simulink model "gm_uz_ssi_interface_2025b"  (R2025b)
settings: Solver=FixedStepDiscrete  StartTime=0.0  StopTime=0.005  RelTol=1e-3
undefined symbols (not defined in the file or in its folder): binary_or_gray, bit_sum, delay_first_clk_on_off, f_ADC, f_clock, PLL, ssi_clk_divider, ssi_encoder_bit_width_multi_turn, ssi_encoder_bit_width_single_turn, ssi_encoder_number_of_status_bits, t_ADC, t_clock, XData
libraries: hdlmdlgenlib x104, hdlsllib x90, simulink x33, simulink_extras x7
(part 2 of 4)

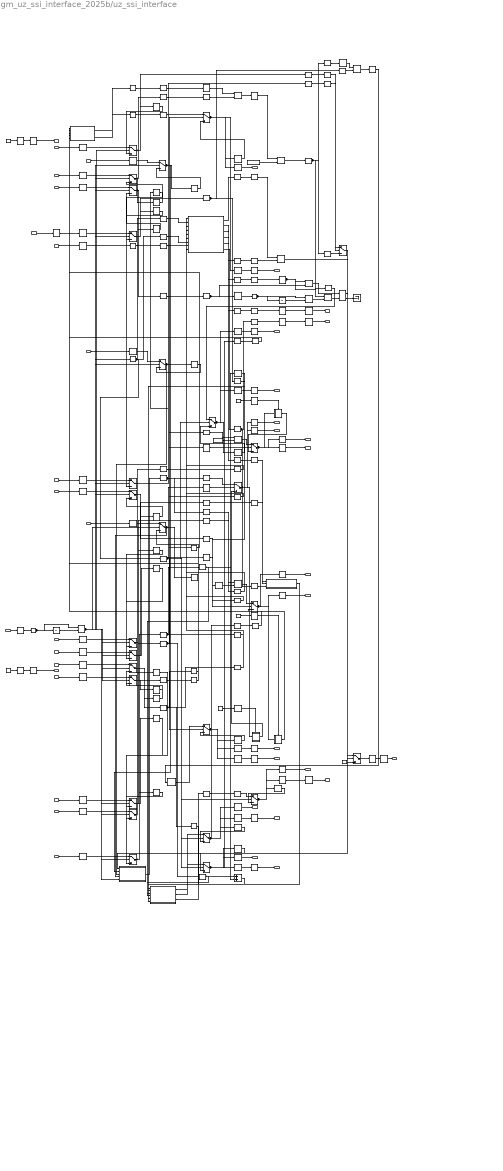
== system gm_uz_ssi_interface_2025b/uz_ssi_interface ==
  note: U(k)
  note: Edge
  note: U(k)
  note: Edge
  note: raw position with encoder offset and aligned wrap for ST and MT position
  note: Processing of raw position data
  note: mech speed SI to el speed SI
  note: decode position and slice data
  note: mech speed SI to el speed SI
  note: SI electrical position
  note: mech speed SI to mech speed RPM
  note: SI mech position to mech speed SI
  note: Acquisition of raw position data from the SSI absolute encoder
  note: ST mech position to SI mech position
  note: pull clk high when disabled
  note: enable logic for clock: turns on and off clk only between transmissions
  ssi_clk_divider_AXI : Inport  OutDataTypeStr=uint32  PortDimensions=1  SampleTime=1e-08
  ssi_encoder_bit_width_single_turn_AXI : Inport  Port=2  OutDataTypeStr=uint32  PortDimensions=1  SampleTime=1e-08
  ssi_encoder_bit_width_multi_turn_AXI : Inport  Port=3  OutDataTypeStr=uint32  PortDimensions=1  SampleTime=1e-08
  ssi_encoder_number_of_status_bits_AXI : Inport  Port=4  OutDataTypeStr=uint32  PortDimensions=1  SampleTime=1e-08
  delay_first_clk_on_off_AXI : Inport  Port=5  OutDataTypeStr=boolean  PortDimensions=1  SampleTime=1e-08
  pos_is_binary_or_gray_AXI : Inport  Port=6  OutDataTypeStr=boolean  PortDimensions=1  SampleTime=1e-08
  ssi_data_in : Inport  Port=7  OutDataTypeStr=boolean  PortDimensions=1  SampleTime=1e-08
  ssi_com_enable_AXI : Inport  Port=8  OutDataTypeStr=boolean  PortDimensions=1  SampleTime=1e-08
  trigger_ssi_read : Inport  Port=9  OutDataTypeStr=boolean  PortDimensions=1  SampleTime=1e-08
  reciprocal_bit_width_single_turn_AXI : Inport  Port=10  OutDataTypeStr=fixdt(0, 27, 27)  PortDimensions=1  SampleTime=1e-08
  t_sample_AXI : Inport  Port=11  OutDataTypeStr=fixdt(0, 18, 24)  PortDimensions=1  SampleTime=1e-08
  kp_pll_AXI : Inport  Port=12  OutDataTypeStr=fixdt(0, 18, 5)  PortDimensions=1  SampleTime=1e-08
  ki_pll_AXI : Inport  Port=13  OutDataTypeStr=fixdt(0, 18, 0)  PortDimensions=1  SampleTime=1e-08
  debug_off_on_AXI : Inport  Port=14  OutDataTypeStr=boolean  PortDimensions=1  SampleTime=1e-08
  position_mech_SI_debug_in_AXI : Inport  Port=15  OutDataTypeStr=fixdt(0, 27, 24)  PortDimensions=1  SampleTime=1e-08
  machine_polepairs_AXI : Inport  Port=16  OutDataTypeStr=uint32  PortDimensions=1  SampleTime=1e-08
  position_mech_offset_ticks_AXI : Inport  Port=17  OutDataTypeStr=int32  PortDimensions=1  SampleTime=1e-08
  sampling_delay_clk_ticks_AXI : Inport  Port=18  OutDataTypeStr=uint32  PortDimensions=1  SampleTime=1e-08
  AND : Logic  AllPortsSameDT=off  OutDataTypeStr=boolean  SampleTime=1e-08
  AND1 : Logic  AllPortsSameDT=off  OutDataTypeStr=boolean  SampleTime=1e-08
  Constant : Constant  Value=6.283172607421875  OutDataTypeStr=fixdt(0, 18, 15)  SampleTime=1e-08
  Constant1 : Constant  OutDataTypeStr=boolean  SampleTime=1e-08
  Constant3 : Constant  Value=0  OutDataTypeStr=boolean  SampleTime=1e-08
  Constant4 : Constant  Value=9.54931640625  OutDataTypeStr=fixdt(0, 18, 14)  SampleTime=1e-08
  Constant5 : Constant  OutDataTypeStr=boolean  SampleTime=1e-08
  Data Type Conversion : DataTypeConversion  OutDataTypeStr=uint8  SampleTime=1e-08  SaturateOnIntegerOverflow=off  RndMeth=Floor
  Data Type Conversion1 : DataTypeConversion  OutDataTypeStr=int32  SampleTime=1e-08  SaturateOnIntegerOverflow=off  RndMeth=Floor
  Delay{,4..5,7..8,10..11,13,15..20,22,24,26..27,29,33..34,37,39..43,46,48,50..52,54..58,62,127,129} (40 alike) : Delay  DelayLength=double(1)  InitialCondition=0  SampleTime=1e-08
  Delay Input1 : UnitDelay  SampleTime=1e-08
  Delay Input11 : UnitDelay  SampleTime=1e-08
  Delay1 : Delay  DelayLength=double(1)  InitialCondition=13  SampleTime=1e-08
  Delay{2..3,6,9,12,21,23,25,28,30,32,36,38,45,47,49,53,64} (18 alike) : Delay  DelayLength=double(2)  InitialCondition=0  SampleTime=1e-08
  Delay14 : Delay  DelayLength=double(1)  InitialCondition=1  SampleTime=1e-08
  Delay31 : Delay  DelayLength=double(1)  InitialCondition=25  SampleTime=1e-08
  Delay35 : Delay  DelayLength=double(1)  InitialCondition=1  SampleTime=1e-08
  Delay44 : Delay  DelayLength=double(1)  InitialCondition=12  SampleTime=1e-08
  Delay59_controlled : Subsystem
  Delay60_controlled : Subsystem
  Delay61_controlled : Subsystem
  FixPt Relational Operator : RelationalOperator  Operator=>  OutDataTypeStr=boolean  SampleTime=1e-08  InputSameDT=off
  FixPt Relational Operator1 : RelationalOperator  Operator=>  OutDataTypeStr=boolean  SampleTime=1e-08  InputSameDT=off
  From{,1..14,16..25,27..32,35..40,42..45} (41 alike) : hdlmdlgenlib/Buffer
  Goto{,1,3..12,14..29} (28 alike) : hdlmdlgenlib/Buffer
  Gray_code_to_binary : Subsystem
  NOT : Logic  Operator=NOT  Inputs=1  AllPortsSameDT=off  OutDataTypeStr=boolean  SampleTime=1e-08
  NOT1 : Logic  Operator=NOT  Inputs=1  AllPortsSameDT=off  OutDataTypeStr=boolean  SampleTime=1e-08
  OR : Logic  Operator=OR  AllPortsSameDT=off  OutDataTypeStr=boolean  SampleTime=1e-08
  Positive : simulink/Logic and Bit Operations/Compare To Constant  relop=>  const=double(0)  OutDataTypeStr=boolean
  Positive1 : simulink/Logic and Bit Operations/Compare To Constant  relop=>  const=double(0)  OutDataTypeStr=boolean
  Product : Product  Inputs=**  OutDataTypeStr=fixdt(0, 27, 24)  SampleTime=1e-08
  Product1 : Product  Inputs=**  OutDataTypeStr=fixdt(1, 27, 12)  SampleTime=1e-08
  Product2 : Product  Inputs=**  OutDataTypeStr=fixdt(1, 27, 12)  SampleTime=1e-08
  Product4 : Product  Inputs=**  OutDataTypeStr=fixdt(0, 27, 20)  SampleTime=1e-08
  Product7 : Product  Inputs=**  OutDataTypeStr=fixdt(0, 27, 24)  SampleTime=1e-08
  S-R Flip-Flop1 : simulink_extras/Flip Flops/S-R Flip-Flop  initial_condition=0
  S-R Flip-Flop1_inst_term1 : Terminator
  Sum2 : Sum  OutDataTypeStr=int32  AccumDataTypeStr=fixdt(0, 33, 0)  SampleTime=1e-08
  Switch{1,6,13,15..16,19..21,31} (9 alike) : Switch  Criteria=u2 > Threshold  Threshold="fi(0,0,1,0,\"hex\",\"0\")"  OutDataTypeStr=uint32  SampleTime=1e-08  SaturateOnIntegerOverflow=off  InputSameDT=off
  Switch{9..10,22,26} (4 alike) : Switch  Criteria=u2 > Threshold  Threshold="fi(0,0,1,0,\"hex\",\"0\")"  OutDataTypeStr=fixdt(0, 27, 24)  SampleTime=1e-08  SaturateOnIntegerOverflow=off  InputSameDT=off
  Switch11 : Switch  Criteria=u2 > Threshold  Threshold="fi(0,0,1,0,\"hex\",\"0\")"  OutDataTypeStr=uint8  SampleTime=1e-08  SaturateOnIntegerOverflow=off  InputSameDT=off
  Switch12 : Switch  Criteria=u2 > Threshold  Threshold="fi(0,0,1,0,\"hex\",\"0\")"  OutDataTypeStr=int32  SampleTime=1e-08  SaturateOnIntegerOverflow=off  InputSameDT=off
  Switch{5,8,14,17..18} (5 alike) : Switch  Criteria=u2 > Threshold  Threshold="fi(0,0,1,0,\"hex\",\"0\")"  OutDataTypeStr=boolean  SampleTime=1e-08  SaturateOnIntegerOverflow=off  InputSameDT=off
  Switch2 : Switch  Criteria=u2 > Threshold  Threshold="fi(0,0,1,0,\"hex\",\"0\")"  OutDataTypeStr=fixdt(0, 27, 27)  SampleTime=1e-08  SaturateOnIntegerOverflow=off  InputSameDT=off
  Switch23 : Switch  Criteria=u2 > Threshold  Threshold="fi(0,0,1,0,\"hex\",\"0\")"  OutDataTypeStr=fixdt(1, 27, 16)  SampleTime=1e-08  SaturateOnIntegerOverflow=off  InputSameDT=off
  Switch24 : Switch  Criteria=u2 > Threshold  Threshold="fi(0,0,1,0,\"hex\",\"0\")"  OutDataTypeStr=fixdt(1, 27, 12)  SampleTime=1e-08  SaturateOnIntegerOverflow=off  InputSameDT=off
  Switch25 : Switch  Criteria=u2 > Threshold  Threshold="fi(0,0,1,0,\"hex\",\"0\")"  OutDataTypeStr=fixdt(1, 27, 12)  SampleTime=1e-08  SaturateOnIntegerOverflow=off  InputSameDT=off
  Switch3 : Switch  Criteria=u2 > Threshold  Threshold="fi(0,0,1,0,\"hex\",\"0\")"  OutDataTypeStr=fixdt(0, 18, 24)  SampleTime=1e-08  SaturateOnIntegerOverflow=off  InputSameDT=off
  Switch4 : Switch  Criteria=u2 > Threshold  Threshold="fi(0,0,1,0,\"hex\",\"0\")"  OutDataTypeStr=fixdt(0, 18, 5)  SampleTime=1e-08  SaturateOnIntegerOverflow=off  InputSameDT=off
  Switch7 : Switch  Criteria=u2 > Threshold  Threshold="fi(0,0,1,0,\"hex\",\"0\")"  OutDataTypeStr=fixdt(0, 18, 0)  SampleTime=1e-08  SaturateOnIntegerOverflow=off  InputSameDT=off
  delayMatch{,1..23} (24 alike) : Delay  DelayLength=double(1)  InitialCondition=0  SampleTime=1e-08
  position_to_speed_pll : Subsystem
  set_offset_to_raw_position_and_wrap : Subsystem
  slice_position_and_status : Subsystem
  ssi_communication : Subsystem
  stateControl : Constant  OutDataTypeStr=boolean  SampleTime=1e-08
  stateControl1 : Constant  OutDataTypeStr=boolean  SampleTime=1e-08
  stateControl2 : Constant  OutDataTypeStr=boolean  SampleTime=1e-08
  wrap_2pi : Subsystem
  ssi_clk : Outport  SampleTime=1e-08
  RW_clk : Outport  Port=2  SampleTime=1e-08
  RW_data : Outport  Port=3  SampleTime=1e-08
  ssi_transaction_done : Outport  Port=4  OutDataTypeStr=boolean  SampleTime=1e-08  LockScale=on
  position_raw_single_turn : Outport  Port=5  OutDataTypeStr=uint32  SampleTime=1e-08  LockScale=on
  position_raw_single_turn_AXI : Outport  Port=6  OutDataTypeStr=uint32  SampleTime=1e-08  LockScale=on
  position_raw_multi_turn : Outport  Port=7  OutDataTypeStr=uint32  SampleTime=1e-08  LockScale=on
  position_raw_multi_turn_AXI : Outport  Port=8  OutDataTypeStr=uint32  SampleTime=1e-08  LockScale=on
  status_raw : Outport  Port=9  OutDataTypeStr=uint32  SampleTime=1e-08  LockScale=on
  status_raw_AXI : Outport  Port=10  OutDataTypeStr=uint32  SampleTime=1e-08  LockScale=on
  ssi_data_out_SH : Outport  Port=11  SampleTime=1e-08
  position_mech_SI_single_turn : Outport  Port=12  SampleTime=1e-08
  position_mech_SI_single_turn_AXI : Outport  Port=13  SampleTime=1e-08
  position_el_SI : Outport  Port=14  SampleTime=1e-08
  position_el_SI_AXI : Outport  Port=15  SampleTime=1e-08
  position_multi_turn : Outport  Port=16  OutDataTypeStr=uint32  SampleTime=1e-08  LockScale=on
  position_multi_turn_AXI : Outport  Port=17  OutDataTypeStr=uint32  SampleTime=1e-08  LockScale=on
  speed_mech_SI : Outport  Port=18  SampleTime=1e-08
  speed_mech_SI_AXI : Outport  Port=19  SampleTime=1e-08
  speed_el_SI : Outport  Port=20  SampleTime=1e-08
  speed_el_SI_AXI : Outport  Port=21  SampleTime=1e-08
  speed_mech_rpm : Outport  Port=22  SampleTime=1e-08
  speed_mech_rpm_AXI : Outport  Port=23  SampleTime=1e-08
  wires:
  Goto24/1 -> From5/1
  Delay53/1 -> Switch18/1
  Switch31/1 -> Delay31/1, Goto7/1
  Delay38/1 -> Switch12/1
  Delay Input11/1 -> FixPt Relational Operator1/2
  Delay12/1 -> Switch20/1
  Delay13/1 -> Switch21/3
  delayMatch14/1 -> position_raw_multi_turn_AXI/1
  Switch21/1 -> delayMatch22/1, Delay13/1, Delay41/1
  Data Type Conversion/1 -> Switch11/1
  From13/1 -> Switch9/1
  delayMatch8/1 -> RW_clk/1
  Delay9/1 -> Switch2/1
  Delay14/1 -> Switch5/3
  Delay41/1 -> delayMatch23/1
  Delay42/1 -> delayMatch21/1
  Positive1/1 -> FixPt Relational Operator1/1, Delay Input11/1
  slice_position_and_status/2(pos_raw_mt) -> Switch16/1
  From19/1 -> Switch9/3
  Switch9/1 -> position_to_speed_pll/1(position_mech_SI)
  Delay30/1 -> Switch10/1
  Delay Input1/1 -> FixPt Relational Operator/2
  Switch26/1 -> Delay42/1, Delay40/1, Delay62/1
  delayMatch1/1 -> Switch23/2
  Goto4/1 -> From42/1
  Delay47/1 -> Switch14/1
  Delay46/1 -> Switch14/3
  Delay49/1 -> Switch15/1
  Positive/1 -> FixPt Relational Operator/1, Delay Input1/1
  Delay22/1 -> Switch4/3
  Switch4/1 -> Delay22/1, position_to_speed_pll/3(kp_pll)
  Product2/1 -> Switch24/1
  Product1/1 -> Switch25/1
  Goto8/1 -> From11/1
  Delay28/1 -> Switch8/1
  From24/1 -> ssi_communication/4(In4)
  delayMatch/1 -> Delay59_controlled/Enable
  OR/1 -> Switch17/1
  ki_pll_AXI/1 -> Delay25/1
  Gray_code_to_binary/1(ssi_pos_binary) -> slice_position_and_status/1(data)
  Delay23/1 -> Switch4/1
  ssi_communication/5(ssi_data_out) -> Goto19/1
  Switch24/1 -> Delay60_controlled/1(in0), Delay56/1, Delay57/1
  Delay59_controlled/1(out0) -> Switch23/3
  FixPt Relational Operator1/1 -> Switch7/2, Switch4/2, Goto22/1, Switch13/2, Switch5/2, Switch20/2, Switch14/2, Switch11/2, Switch2/2, Switch10/2, Switch8/2, Switch1/2, Switch3/2, Switch15/2, position_to_speed_pll/5(Trigger), Switch12/2, Switch31/2, Switch18/2
  Delay24/1 -> Switch7/3
  From30/1 -> Switch19/1
  debug_off_on_AXI/1 -> Delay28/1
  Delay44/1 -> Switch13/3
  Delay25/1 -> Switch7/1
  Goto21/1 -> From18/1
  Delay40/1 -> delayMatch20/1
  From10/1 -> delayMatch1/1, Switch6/2, Switch22/2, Switch26/2, delayMatch6/1, Switch21/2, Switch19/2, delayMatch4/1, Switch16/2
  From28/1 -> NOT/1
  Delay11/1 -> delayMatch19/1
  Delay33/1 -> speed_mech_rpm/1
  Goto15/1 -> From43/1, From35/1, From24/1
  FixPt Relational Operator/1 -> AND1/2
  Delay21/1 -> Switch3/1
  Delay10/1 -> delayMatch18/1
  delayMatch11/1 -> position_raw_single_turn/1
  Delay20/1 -> Switch3/3
  Delay29/1 -> Switch10/3
  Goto22/1 -> From38/1, From39/1, From10/1
  Goto3/1 -> From7/1
  Delay4/1 -> delayMatch8/1
  delayMatch20/1 -> position_el_SI/1
  wrap_2pi/1(output) -> Switch26/1
  Delay55/1 -> delayMatch16/1
  Delay51/1 -> delayMatch14/1
  Delay15/1 -> Switch6/3
  Switch13/1 -> Goto15/1, Delay44/1
  stateControl1/1 -> delayMatch3/1
  Switch19/1 -> delayMatch15/1, Delay54/1, Delay55/1
  delayMatch13/1 -> position_raw_multi_turn/1
  Goto9/1 -> From25/1, From37/1
  Delay5/1 -> Switch20/3
  Delay6/1 -> Switch5/1
  From37/1 -> slice_position_and_status/4(bit_width_status), Sum2/2, Data Type Conversion1/1
  Switch8/1 -> Goto8/1, Delay27/1
  Goto/1 -> From23/1, From44/1, From36/1
  Delay31/1 -> Switch31/3
  Delay45/1 -> Switch13/1
  Delay2/1 -> Switch1/1
  slice_position_and_status/3(raw_status) -> Goto20/1
  Delay64/1 -> Switch31/1
  Delay17/1 -> delayMatch17/1
  Delay16/1 -> delayMatch12/1
  Product4/1 -> Delay43/1
  position_mech_offset_ticks_AXI/1 -> Delay38/1
  Delay129/1 -> delayMatch10/1
  Delay7/1 -> delayMatch9/1
  Goto28/1 -> From12/1
  stateControl/1 -> delayMatch/1
  Delay127/1 -> delayMatch7/1
  stateControl2/1 -> delayMatch5/1
  Delay34/1 -> speed_mech_rpm_AXI/1
  delay_first_clk_on_off_AXI/1 -> Delay6/1
  Delay57/1 -> speed_el_SI_AXI/1
  Delay56/1 -> speed_el_SI/1
  Switch14/1 -> Delay46/1, Goto16/1
  Delay18/1 -> speed_mech_SI_AXI/1
  Delay19/1 -> speed_mech_SI/1
  delayMatch10/1 -> ssi_transaction_done/1
  delayMatch23/1 -> position_multi_turn_AXI/1
  delayMatch21/1 -> position_el_SI_AXI/1
  Switch22/1 -> Delay10/1, Delay58/1, Delay11/1
  delayMatch19/1 -> position_mech_SI_single_turn_AXI/1
  delayMatch18/1 -> position_mech_SI_single_turn/1
  delayMatch17/1 -> ssi_data_out_SH/1
  From12/1 -> Switch21/1
  delayMatch16/1 -> status_raw_AXI/1
  delayMatch12/1 -> position_raw_single_turn_AXI/1
  delayMatch9/1 -> RW_data/1
  delayMatch7/1 -> ssi_clk/1
  set_offset_to_raw_position_and_wrap/1(st_raw_with_offset_and_wrapped) -> Goto29/1
  Goto5/1 -> From6/1
  Delay43/1 -> wrap_2pi/1(input)
  machine_polepairs_AXI/1 -> Delay36/1
  Goto27/1 -> From45/1
  Goto23/1 -> From40/1
  Goto7/1 -> From4/1
  Goto20/1 -> From30/1
  ssi_communication/1(ssi_clk) -> Goto24/1
  Goto19/1 -> From29/1
  Switch5/1 -> Delay14/1, Goto1/1
  Delay39/1 -> Product4/1
  delayMatch2/1 -> Product2/2
  Goto6/1 -> From28/1
  Goto18/1 -> From27/1
  Goto26/1 -> From20/1
  Goto29/1 -> From2/1
  Goto10/1 -> From13/1
  Goto1/1 -> From1/1
  ssi_communication/6(ssi_transaction_done) -> Goto17/1
  Constant/1 -> Product7/2
  ssi_communication/4(ssi_data_raw) -> Goto21/1
  S-R Flip-Flop1/1 -> Switch17/2
  ssi_communication/3(ssi_clk_idle_levels) -> Goto23/1
  ssi_communication/2(ssi_clk_enb_out) -> Goto6/1
  Goto14/1 -> From21/1, From19/1, From22/1
  slice_position_and_status/1(pos_raw_st) -> Switch6/1
  set_offset_to_raw_position_and_wrap/2(mt_raw_with_offset_and_wrapped) -> Goto28/1
  From7/1 -> ssi_communication/8(ssi_data_in)
  Constant1/1 -> Delay4/1
  position_to_speed_pll/1(speed_mech_SI) -> Goto12/1
  ssi_com_enable_AXI/1 -> Delay53/1
  From36/1 -> slice_position_and_status/3(bit_width_st), Sum2/1
  delayMatch22/1 -> position_multi_turn/1
  Switch15/1 -> Delay48/1, Goto9/1
  delayMatch15/1 -> status_raw/1
  ssi_data_in/1 -> Delay3/1
  Constant3/1 -> Delay7/1
  Switch17/1 -> Delay127/1
  From27/1 -> AND/2, NOT1/1
  S-R Flip-Flop1/2 -> S-R Flip-Flop1_inst_term1/1
  Product7/1 -> Goto14/1
  From9/1 -> ssi_communication/9(sampling_delay_clk_ticks)
  Product/1 -> Delay26/1
  Switch16/1 -> delayMatch13/1, Goto26/1, Delay50/1, Delay51/1
  NOT1/1 -> Positive/1
  From8/1 -> Gray_code_to_binary/3(trigger)
  From6/1 -> Product/2
  AND/1 -> S-R Flip-Flop1/1
  From5/1 -> OR/1
  From40/1 -> OR/2
  ssi_clk_divider_AXI/1 -> Delay64/1
  From39/1 -> ssi_communication/7(trigger_ssi)
  From38/1 -> ssi_communication/2(ssi_clk_reset)
  From31/1 -> Product2/1
  From3/1 -> Switch23/1
  t_sample_AXI/1 -> Delay21/1
  Delay/1 -> Product/1
  From29/1 -> Delay17/1
  Switch25/1 -> Delay61_controlled/1(in0), Delay34/1, Delay33/1
  From22/1 -> Delay39/1
  From2/1 -> Delay/1
  From18/1 -> Gray_code_to_binary/1(ssi_data_raw)
  From17/1 -> Gray_code_to_binary/2(pos_is_binary_or_gray)
  From16/1 -> Product4/2
  From14/1 -> Product1/1
  From11/1 -> Switch9/2
  From1/1 -> ssi_communication/6(delay_first_clk_on_off)
  ssi_encoder_number_of_status_bits_AXI/1 -> Delay49/1
  From/1 -> Delay129/1
  Constant4/1 -> Product1/2
  Delay36/1 -> Data Type Conversion/1
  Delay32/1 -> Positive1/1
  Delay3/1 -> Goto3/1
  sampling_delay_clk_ticks_AXI/1 -> Delay12/1
  Delay26/1 -> Product7/1
  Constant5/1 -> Switch17/3
  Switch6/1 -> Goto4/1, Delay16/1, Delay15/1, delayMatch11/1
  AND1/1 -> S-R Flip-Flop1/2
  position_mech_SI_debug_in_AXI/1 -> Delay30/1
  kp_pll_AXI/1 -> Delay23/1
  reciprocal_bit_width_single_turn_AXI/1 -> Delay9/1
  trigger_ssi_read/1 -> Delay32/1
  pos_is_binary_or_gray_AXI/1 -> Delay47/1
  ssi_encoder_bit_width_multi_turn_AXI/1 -> Delay45/1
  ssi_encoder_bit_width_single_turn_AXI/1 -> Delay2/1
  Switch23/1 -> Delay59_controlled/1(in0), Delay19/1, Delay18/1
  Goto12/1 -> From31/1, From14/1, From3/1
  Sum2/1 -> slice_position_and_status/5(shift_val_mt)
  Goto11/1 -> From16/1, From32/1
  Goto17/1 -> From8/1, From/1
  Switch7/1 -> position_to_speed_pll/4(ki_pll), Delay24/1
  Switch3/1 -> position_to_speed_pll/2(t_sample), Delay20/1
  Switch20/1 -> Goto25/1, Delay5/1
  Switch2/1 -> Goto5/1, Delay8/1
  Switch18/1 -> Goto18/1, Delay52/1
  Switch1/1 -> Goto/1, Delay1/1
  Switch12/1 -> Goto27/1, Delay37/1
  NOT/1 -> AND1/1, AND/1
  Switch11/1 -> Goto11/1, Delay35/1
  Switch10/1 -> Goto10/1, Delay29/1
  Delay52/1 -> Switch18/3
  delayMatch6/1 -> Switch25/2
  Goto25/1 -> From9/1
  Goto16/1 -> From17/1
  delayMatch4/1 -> Switch24/2
  Delay8/1 -> Switch2/3
  delayMatch3/1 -> Delay60_controlled/Enable
  delayMatch5/1 -> Delay61_controlled/Enable
  Delay27/1 -> Switch8/3
  Data Type Conversion1/1 -> slice_position_and_status/6(shift_val_st)
  Delay1/1 -> Switch1/3
  Delay37/1 -> Switch12/3
  Delay60_controlled/1(out0) -> Switch24/3
  Delay50/1 -> Switch16/3
  From43/1 -> set_offset_to_raw_position_and_wrap/5(n1)
  Delay61_controlled/1(out0) -> Switch25/3
  Delay35/1 -> Switch11/3
  Delay48/1 -> Switch15/3
  Delay54/1 -> Switch19/3
  Delay58/1 -> Switch22/3
  Delay62/1 -> Switch26/3
  From4/1 -> ssi_communication/1(ssi_clk_divider)
  From20/1 -> set_offset_to_raw_position_and_wrap/1(mt_raw)
  From21/1 -> Switch22/1
  From25/1 -> ssi_communication/5(In5)
  From23/1 -> ssi_communication/3(In3)
  From44/1 -> set_offset_to_raw_position_and_wrap/2(n)
  From32/1 -> delayMatch2/1
  From35/1 -> slice_position_and_status/2(bit_width_mt)
  From42/1 -> set_offset_to_raw_position_and_wrap/3(st_raw)
  From45/1 -> set_offset_to_raw_position_and_wrap/4(In4)

== system gm_uz_ssi_interface_2025b/uz_ssi_interface/Delay59_controlled ==
  in0 : Inport  OutDataTypeStr=fixdt(1, 27, 16)  SampleTime=1e-08
  stateControl : EnablePort  OutDataTypeStr=boolean
  Delay59 : Delay  DelayLength=double(1)  InitialCondition=0  SampleTime=1e-08
  out0 : Outport  OutDataTypeStr=fixdt(1, 27, 16)  SampleTime=1e-08
  wires:
  in0/1 -> Delay59/1
  Delay59/1 -> out0/1

== system gm_uz_ssi_interface_2025b/uz_ssi_interface/Delay60_controlled ==
  in0 : Inport  OutDataTypeStr=fixdt(1, 27, 12)  SampleTime=1e-08
  stateControl : EnablePort  OutDataTypeStr=boolean
  Delay60 : Delay  DelayLength=double(1)  InitialCondition=0  SampleTime=1e-08
  out0 : Outport  OutDataTypeStr=fixdt(1, 27, 12)  SampleTime=1e-08
  wires:
  in0/1 -> Delay60/1
  Delay60/1 -> out0/1

== system gm_uz_ssi_interface_2025b/uz_ssi_interface/Delay61_controlled ==
  in0 : Inport  OutDataTypeStr=fixdt(1, 27, 12)  SampleTime=1e-08
  stateControl : EnablePort  OutDataTypeStr=boolean
  Delay61 : Delay  DelayLength=double(1)  InitialCondition=0  SampleTime=1e-08
  out0 : Outport  OutDataTypeStr=fixdt(1, 27, 12)  SampleTime=1e-08
  wires:
  in0/1 -> Delay61/1
  Delay61/1 -> out0/1

== system gm_uz_ssi_interface_2025b/uz_ssi_interface/Gray_code_to_binary ==
  ssi_data_raw : Inport  OutDataTypeStr=fixdt(0, 64, 0)  PortDimensions=1  SampleTime=1e-08
  pos_is_binary_or_gray : Inport  Port=2  OutDataTypeStr=boolean  PortDimensions=1  SampleTime=1e-08
  trigger : Inport  Port=3  OutDataTypeStr=boolean  PortDimensions=1  SampleTime=1e-08
  Delay : Delay  DelayLength=double(1)  InitialCondition=0  SampleTime=1e-08
  Delay2 : Delay  DelayLength=double(101)  InitialCondition=0  SampleTime=1e-08
  Delay6 : Delay  DelayLength=double(1)  InitialCondition=0  SampleTime=1e-08
  Switch : Switch  Criteria=u2 > Threshold  Threshold="fi(0,0,1,0,\"hex\",\"0\")"  OutDataTypeStr=fixdt(0, 64, 0)  SampleTime=1e-08  SaturateOnIntegerOverflow=off  InputSameDT=off
  gray_to_bin : Subsystem
  ssi_pos_binary : Outport  SampleTime=1e-08
  wires:
  ssi_data_raw/1 -> Delay/1, Delay2/1
  trigger/1 -> gray_to_bin/2(enb)
  Delay/1 -> gray_to_bin/1(gray)
  gray_to_bin/1(binary_out) -> Delay6/1
  pos_is_binary_or_gray/1 -> Switch/2
  Delay2/1 -> Switch/3
  Delay6/1 -> Switch/1
  Switch/1 -> ssi_pos_binary/1

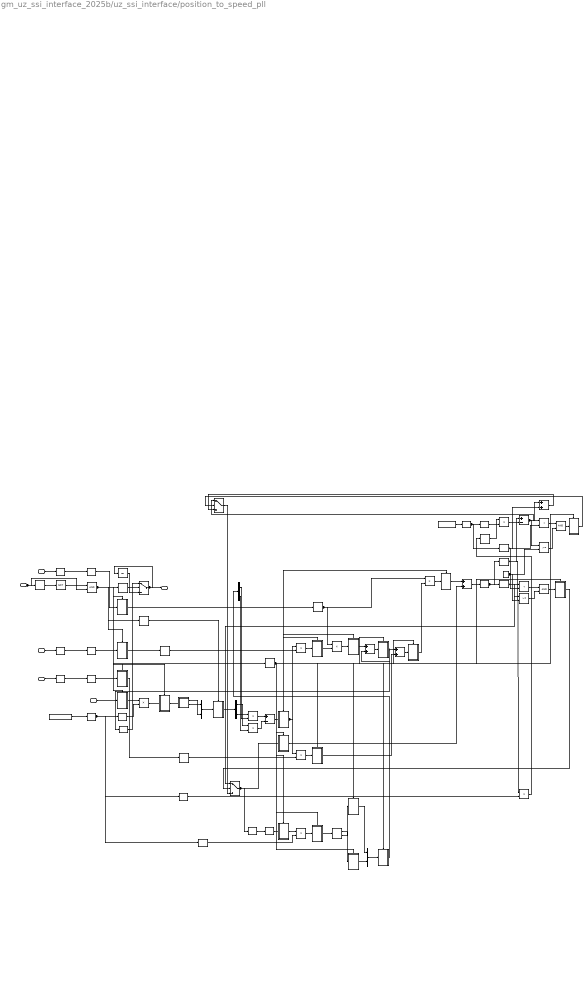
== system gm_uz_ssi_interface_2025b/uz_ssi_interface/position_to_speed_pll ==
  note: pi_controller
  note: +/- 198000
  note: -2 ... 2
  note: wrap 2pi
  note: <<1
  note: phase discriminator
  note: -1 ... 1
  note: pll
  note: -1 ... 1
  note: integrator
  note: 20
  note: +/- 1300
  note: remainder
  position_mech_SI : Inport  OutDataTypeStr=fixdt(0, 27, 24)  PortDimensions=1  SampleTime=1e-08
  t_sample : Inport  Port=2  OutDataTypeStr=fixdt(0, 18, 24)  PortDimensions=1  SampleTime=1e-08
  kp_pll : Inport  Port=3  OutDataTypeStr=fixdt(0, 18, 5)  PortDimensions=1  SampleTime=1e-08
  ki_pll : Inport  Port=4  OutDataTypeStr=fixdt(0, 18, 0)  PortDimensions=1  SampleTime=1e-08
  Trigger : Inport  Port=5  OutDataTypeStr=boolean  SampleTime=1e-08
  AND : Logic  AllPortsSameDT=off  OutDataTypeStr=boolean  SampleTime=1e-08
  AND1 : Logic  AllPortsSameDT=off  OutDataTypeStr=boolean  SampleTime=1e-08
  Constant1 : Constant  Value=0.1591548919677734375  OutDataTypeStr=fixdt(0, 18, 20)  SampleTime=1e-08
  Constant7 : Constant  Value=0  OutDataTypeStr=fixdt(0, 27, 24)  SampleTime=1e-08
  Constant8 : Constant  Value=6.283172607421875  OutDataTypeStr=fixdt(0, 18, 15)  SampleTime=1e-08
  Delay : Subsystem
      settings: MinAlgLoopOccurrences=on
  Delay1 : Subsystem
      settings: MinAlgLoopOccurrences=on
  Delay10 : Subsystem
      settings: MinAlgLoopOccurrences=on
  Delay11 : Subsystem
      settings: MinAlgLoopOccurrences=on
  Delay12 : Subsystem
      settings: MinAlgLoopOccurrences=on
  Delay13 : Subsystem
      settings: MinAlgLoopOccurrences=on
  Delay14 : Subsystem
      settings: MinAlgLoopOccurrences=on
  Delay18 : Subsystem
      settings: MinAlgLoopOccurrences=on
  Delay19 : Subsystem
      settings: MinAlgLoopOccurrences=on
  Delay2 : Subsystem
      settings: MinAlgLoopOccurrences=on
  Delay20 : Subsystem
      settings: MinAlgLoopOccurrences=on
  Delay21 : Subsystem
      settings: MinAlgLoopOccurrences=on
  Delay22 : Subsystem
      settings: MinAlgLoopOccurrences=on
  Delay23 : Subsystem
      settings: MinAlgLoopOccurrences=on
  Delay3 : Subsystem
      settings: MinAlgLoopOccurrences=on
  Delay4 : Subsystem
      settings: MinAlgLoopOccurrences=on
  Delay5 : Subsystem
      settings: MinAlgLoopOccurrences=on
  Delay6 : Subsystem
      settings: MinAlgLoopOccurrences=on
  Delay7 : Subsystem
      settings: MinAlgLoopOccurrences=on
  Delay8 : Subsystem
      settings: MinAlgLoopOccurrences=on
  Delay9 : Subsystem
      settings: MinAlgLoopOccurrences=on
  From{,1..6,11,13..15} (11 alike) : hdlmdlgenlib/Buffer
  Goto{,1..3,8,10..11} (7 alike) : hdlmdlgenlib/Buffer
  Product1 : Product  Inputs=**  OutDataTypeStr=fixdt(1, 27, 23)  SampleTime=1e-08
  Product10 : Product  Inputs=**  OutDataTypeStr=fixdt(1, 27, 20)  SampleTime=1e-08
  Product2 : Product  Inputs=**  OutDataTypeStr=fixdt(1, 27, 25)  SampleTime=1e-08
  Product3 : Product  Inputs=**  OutDataTypeStr=fixdt(1, 27, 25)  SampleTime=1e-08
  Product4 : Product  Inputs=**  OutDataTypeStr=fixdt(1, 27, 20)  SampleTime=1e-08
  Product5 : Product  Inputs=**  OutDataTypeStr=fixdt(1, 27, 8)  SampleTime=1e-08
  Product6 : Product  Inputs=**  OutDataTypeStr=fixdt(1, 27, 14)  SampleTime=1e-08
  Product7 : Product  Inputs=**  OutDataTypeStr=fixdt(1, 27, 23)  SampleTime=1e-08
  Product8 : Product  Inputs=**  OutDataTypeStr=fixdt(1, 27, 26)  SampleTime=1e-08
  Product9 : Product  Inputs=**  OutDataTypeStr=fixdt(1, 27, 20)  SampleTime=1e-08
  Relational Operator1 : RelationalOperator  Operator=<  OutDataTypeStr=boolean  SampleTime=1e-08  InputSameDT=off
  Relational Operator2 : RelationalOperator  OutDataTypeStr=boolean  SampleTime=1e-08  InputSameDT=off
  Relational Operator3 : RelationalOperator  Operator=<  OutDataTypeStr=boolean  SampleTime=1e-08  InputSameDT=off
  Relational Operator4 : RelationalOperator  OutDataTypeStr=boolean  SampleTime=1e-08  InputSameDT=off
  Sine HDL Optimized : Subsystem  mask(Sine and Cosine HDL optimized block){OutputFormula=sin(2*pi*u) and cos(2*pi*u), NumDataPoints=double(256), TableDataTypeStr=fixdt(0,26,20), SimulateLUTROMDelay=off}
      mask prompts: OutputFormula "Simulink:masks:OutputFormula_MP"; NumDataPoints "HDLShared:hdlshared:CosineHDL_Npts"; TableDataTypeStr "Simulink:blkprm_prompts:TABLE_UNIFIEDDATATYPE"; SimulateLUTROMDelay "HDLShared:hdlshared:CosineHDL_SimulateLUTDelay"
      mask help: Sine and Cosine HDL optimized block using quarter wave symmetry, and HDL friendly settings.
      mask init:
      | NumDataPoints = double(256);
      | OutputFormula = double(4);
      | SampleTime = double(-1);
      | SimulateLUTROMDelay = double(0);
      | TableDataTypeStr = fixdt(0,26,20);
      | curr_blk_name = 'uz_ssi_interface_2025b/uz_ssi_interface/position_to_speed_pll/Sine\nHDL Optimized';
      | sys_name = 'uz_ssi_interface_2025b/uz_ssi_interface/position_to_speed_pll';
      mask Help: helpview([docroot '/hdlcoder/helptargets.map'],'SineAndCosineHDL_Optimized');
      mask TypeOptions OutputFormula: sin(2*pi*u) | cos(2*pi*u) | exp(j*2*pi*u) | sin(2*pi*u) and cos(2*pi*u)
      mask Display:
      | port_label('input',1,'u')
      | port_label('output',1,'sin(2*pi*u)')
      | port_label('output',2,'cos(2*pi*u)')
      | xpos = 0.35;
      | yoffset = 0.5;
      | if ( SimulateLUTROMDelay )
      |   text(xpos,yoffset,'HDL (Z^{-1})','texmode','on')
      | else
      |    text(xpos,yoffset,'HDL')
      | end
  Sine HDL Optimized1 : Subsystem  mask(Sine and Cosine HDL optimized block){OutputFormula=sin(2*pi*u) and cos(2*pi*u), NumDataPoints=double(256), TableDataTypeStr=fixdt(0,26,20), SimulateLUTROMDelay=off}
      mask prompts: OutputFormula "Simulink:masks:OutputFormula_MP"; NumDataPoints "HDLShared:hdlshared:CosineHDL_Npts"; TableDataTypeStr "Simulink:blkprm_prompts:TABLE_UNIFIEDDATATYPE"; SimulateLUTROMDelay "HDLShared:hdlshared:CosineHDL_SimulateLUTDelay"
      mask help: Sine and Cosine HDL optimized block using quarter wave symmetry, and HDL friendly settings.
      mask init:
      | NumDataPoints = double(256);
      | OutputFormula = double(4);
      | SampleTime = double(-1);
      | SimulateLUTROMDelay = double(0);
      | TableDataTypeStr = fixdt(0,26,20);
      | curr_blk_name = 'uz_ssi_interface_2025b/uz_ssi_interface/position_to_speed_pll/Sine\nHDL Optimized1';
      | sys_name = 'uz_ssi_interface_2025b/uz_ssi_interface/position_to_speed_pll';
      mask Help: helpview([docroot '/hdlcoder/helptargets.map'],'SineAndCosineHDL_Optimized');
      mask TypeOptions OutputFormula: sin(2*pi*u) | cos(2*pi*u) | exp(j*2*pi*u) | sin(2*pi*u) and cos(2*pi*u)
      mask Display:
      | port_label('input',1,'u')
      | port_label('output',1,'sin(2*pi*u)')
      | port_label('output',2,'cos(2*pi*u)')
      | xpos = 0.35;
      | yoffset = 0.5;
      | if ( SimulateLUTROMDelay )
      |   text(xpos,yoffset,'HDL (Z^{-1})','texmode','on')
      | else
      |    text(xpos,yoffset,'HDL')
      | end
  Sum1 : Sum  Inputs=+-  OutDataTypeStr=fixdt(1, 27, 24)  AccumDataTypeStr=fixdt(1, 27, 24)  SampleTime=1e-08
  Sum2 : Sum  OutDataTypeStr=fixdt(1, 27, 16)  AccumDataTypeStr=fixdt(1, 32, 20)  SampleTime=1e-08
  Sum3 : Sum  OutDataTypeStr=fixdt(1, 27, 14)  AccumDataTypeStr=fixdt(1, 30, 16)  SampleTime=1e-08
  Sum4 : Sum  OutDataTypeStr=fixdt(1, 27, 23)  AccumDataTypeStr=fixdt(1, 31, 26)  SampleTime=1e-08
  Sum5 : Sum  Inputs=+-  OutDataTypeStr=fixdt(1, 27, 23)  AccumDataTypeStr=fixdt(1, 28, 23)  SampleTime=1e-08
  Sum6 : Sum  OutDataTypeStr=fixdt(1, 27, 23)  AccumDataTypeStr=fixdt(1, 28, 23)  SampleTime=1e-08
  Switch3 : Switch  Criteria=u2 > Threshold  Threshold="fi(0,0,1,0,\"hex\",\"0\")"  OutDataTypeStr=fixdt(1, 27, 23)  SampleTime=1e-08  SaturateOnIntegerOverflow=off  InputSameDT=off
  Switch4 : Switch  Criteria=u2 > Threshold  Threshold="fi(0,0,1,0,\"hex\",\"0\")"  OutDataTypeStr=fixdt(1, 27, 23)  SampleTime=1e-08  SaturateOnIntegerOverflow=off  InputSameDT=off
  Trigger_delay : Delay  DelayLength=double(1)  InitialCondition=0
  Trigger_delayed_inverted_and_Trigger : Logic  AllPortsSameDT=off  OutDataTypeStr=boolean  SampleTime=1e-08
  delayMatch{,1..5} (6 alike) : Delay  DelayLength=double(1)  InitialCondition=0
  fixed_point_floor : Subsystem
  mux : Mux  Inputs=2
  mux1 : Mux  Inputs=2
  not_Trigger_delayed : Logic  Operator=NOT  Inputs=1  AllPortsSameDT=off  OutDataTypeStr=boolean  SampleTime=1e-08
  omega_mechbypassMux : Switch  Criteria=u2 ~= 0  Threshold=double(0)  OutDataTypeStr=fixdt(1, 27, 16)  SampleTime=1e-08  SaturateOnIntegerOverflow=off  InputSameDT=off
  out0_bypass : UnitDelay  InitialCondition="fi(0,1,27,16,\"hex\",\"0000000\")"  SampleTime=1e-08
  t : Demux  Outputs=2
  t1 : Demux  Outputs=2
  t2 : hdlmdlgenlib/Buffer
  speed_mech_SI : Outport  SampleTime=1e-08  InitialOutput=[0]
  wires:
  Goto2/1 -> From2/1
  Delay14/1(out0) -> Sine HDL Optimized1/1(u)
  ki_pll/1 -> Goto2/1
  delayMatch5/1 -> omega_mechbypassMux/2
  Trigger/1 -> Trigger_delayed_inverted_and_Trigger/2, Trigger_delay/1
  Delay3/1(out0) -> Sum3/2
  From4/1 -> Product7/2
  delayMatch/1 -> Delay1/Enable
  t_sample/1 -> Goto/1
  Delay4/1(out0) -> Sum2/1
  Trigger_delay/1 -> not_Trigger_delayed/1
  Trigger_delayed_inverted_and_Trigger/1 -> Delay13/Enable, delayMatch/1, Delay7/Enable, delayMatch1/1, Delay6/Enable, delayMatch5/1, Delay14/Enable, Delay8/Enable
  kp_pll/1 -> Goto1/1
  not_Trigger_delayed/1 -> Trigger_delayed_inverted_and_Trigger/1
  Goto/1 -> From/1
  From3/1 -> Delay11/1(in0)
  Goto1/1 -> From1/1
  Delay5/1(out0) -> Product4/2
  Constant1/1 -> Goto3/1
  omega_mechbypassMux/1 -> out0_bypass/1, speed_mech_SI/1
  out0_bypass/1 -> omega_mechbypassMux/3
  From/1 -> Delay6/1(in0)
  From2/1 -> Delay7/1(in0)
  From1/1 -> Delay8/1(in0)
  Delay1/1(out0) -> t/1
  Delay19/1(out0) -> Sum4/2
  position_mech_SI/1 -> Delay13/1(in0)
  From15/1 -> Sum5/1, Product7/1
  Goto3/1 -> From4/1, From6/1, From5/1
  Sine HDL Optimized1/1(x) -> mux/2
  Delay6/1(out0) -> delayMatch3/1
  Product5/1 -> Delay5/1(in0)
  Delay7/1(out0) -> delayMatch4/1
  Product3/1 -> Sum1/1
  Delay8/1(out0) -> delayMatch2/1
  From13/1 -> Relational Operator3/2, Sum6/2, Relational Operator1/2
  Delay11/1(out0) -> Product9/1
  Delay23/1(out0) -> mux1/1
  Delay13/1(out0) -> Product10/1
  Switch3/1 -> Delay19/1(in0), Goto8/1
  From6/1 -> Product10/2
  t2/1 -> omega_mechbypassMux/1
  Product10/1 -> Delay14/1(in0)
  delayMatch4/1 -> Product5/2
  Sine HDL Optimized1/2(y) -> mux/1
  delayMatch3/1 -> Product8/1, Product4/1
  delayMatch2/1 -> Product6/2
  Delay12/1(out0) -> Sine HDL Optimized/1(u)
  Product2/1 -> Sum1/2
  mux/1 -> Delay1/1(in0)
  From5/1 -> Product9/2
  Switch4/1 -> Switch3/3
  t1/2 -> Product2/2
  t1/1 -> Product3/2
  t/2 -> Product3/1
  t/1 -> Product2/1
  Goto8/1 -> From3/1
  delayMatch1/1 -> Delay2/Enable, Delay11/Enable, Delay9/Enable, Delay10/Enable, Delay18/Enable, Delay5/Enable, Delay4/Enable, Delay20/Enable, Delay21/Enable, Delay22/Enable, Delay23/Enable, Delay19/Enable, Delay3/Enable, Delay/Enable, Delay12/Enable
  Sum1/1 -> Delay2/1(in0)
  Delay2/1(out0) -> Product6/1, Product5/1
  Product6/1 -> Delay3/1(in0)
  Product9/1 -> Delay12/1(in0)
  Sine HDL Optimized/1(x) -> Delay22/1(in0)
  Product4/1 -> Delay4/1(in0)
  Sine HDL Optimized/2(y) -> Delay23/1(in0)
  Delay20/1(out0) -> Switch4/2
  Delay22/1(out0) -> mux1/2
  Sum2/1 -> Delay/1(in0)
  mux1/1 -> Delay18/1(in0)
  Delay/1(out0) -> Sum2/2, t2/1, Sum3/1
  Delay18/1(out0) -> t1/1
  Sum3/1 -> Delay9/1(in0)
  Delay9/1(out0) -> Product8/2
  Product8/1 -> Delay10/1(in0)
  Constant8/1 -> Goto11/1
  Delay10/1(out0) -> Sum4/1
  Goto11/1 -> From13/1, From14/1
  Sum4/1 -> Goto10/1
  From14/1 -> Product1/2
  fixed_point_floor/1(y) -> Product1/1
  Goto10/1 -> From15/1, From11/1
  Product1/1 -> Sum5/2
  Constant7/1 -> Relational Operator4/2, Relational Operator2/2
  From11/1 -> Switch3/1, Relational Operator2/1, Relational Operator1/1
  Sum5/1 -> Switch4/1, Sum6/1, Relational Operator4/1, Relational Operator3/1
  Relational Operator1/1 -> AND/1
  Relational Operator2/1 -> AND/2
  Product7/1 -> fixed_point_floor/1(x)
  Sum6/1 -> Switch4/3
  Relational Operator3/1 -> AND1/1
  Relational Operator4/1 -> AND1/2
  AND/1 -> Delay21/1(in0)
  AND1/1 -> Delay20/1(in0)
  Delay21/1(out0) -> Switch3/2

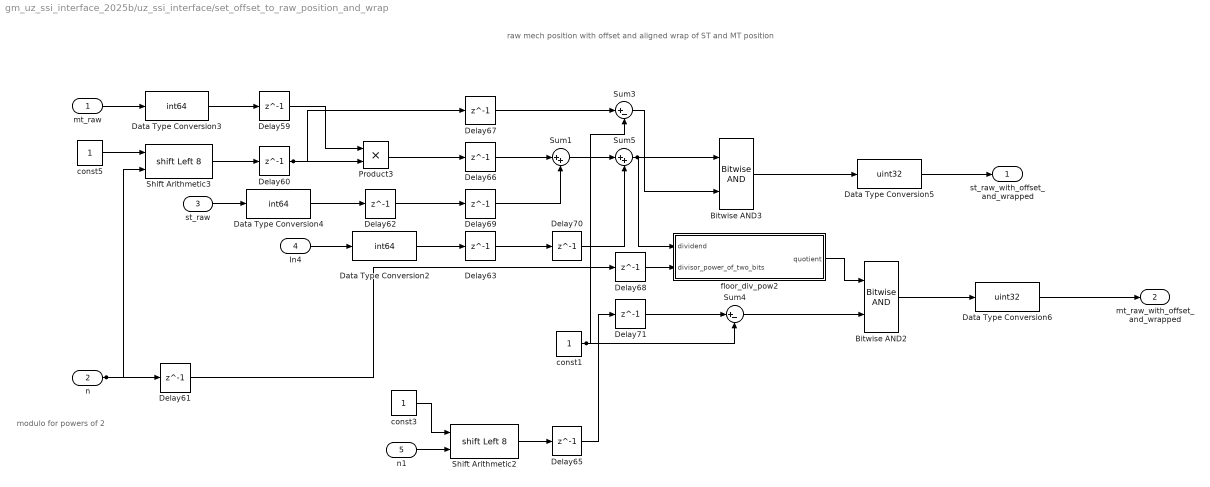
== system gm_uz_ssi_interface_2025b/uz_ssi_interface/set_offset_to_raw_position_and_wrap ==
  note: modulo for powers of 2
  note: raw mech position with offset and aligned wrap of ST and MT position
  mt_raw : Inport  OutDataTypeStr=uint32  PortDimensions=1  SampleTime=1e-08
  n : Inport  Port=2  OutDataTypeStr=uint32  PortDimensions=1  SampleTime=1e-08
  st_raw : Inport  Port=3  OutDataTypeStr=uint32  PortDimensions=1  SampleTime=1e-08
  In4 : Inport  Port=4  OutDataTypeStr=int32  PortDimensions=1  SampleTime=1e-08
  n1 : Inport  Port=5  OutDataTypeStr=uint32  PortDimensions=1  SampleTime=1e-08
  Bitwise AND2 : simulink/Logic and Bit Operations/Bitwise Operator  logicop=AND  UseBitMask=off  NumInputPorts=2  BitMask=bin2dec('11011001')  BitMaskRealWorld=Stored Integer
      settings: LibrarySourceBlock=|
      | simulink/Quick Insert/Logic and Bit
      | Operations/Bitwise AND
  Bitwise AND3 : simulink/Logic and Bit Operations/Bitwise Operator  logicop=AND  UseBitMask=off  NumInputPorts=2  BitMask=bin2dec('11011001')  BitMaskRealWorld=Stored Integer
      settings: LibrarySourceBlock=|
      | simulink/Quick Insert/Logic and Bit
      | Operations/Bitwise AND
  Data Type Conversion2 : DataTypeConversion  OutDataTypeStr=int64  SaturateOnIntegerOverflow=off  RndMeth=Floor
  Data Type Conversion3 : DataTypeConversion  OutDataTypeStr=int64  SaturateOnIntegerOverflow=off  RndMeth=Floor
  Data Type Conversion4 : DataTypeConversion  OutDataTypeStr=int64  SaturateOnIntegerOverflow=off  RndMeth=Floor
  Data Type Conversion5 : DataTypeConversion  OutDataTypeStr=uint32  SaturateOnIntegerOverflow=off  RndMeth=Floor
  Data Type Conversion6 : DataTypeConversion  OutDataTypeStr=uint32  SaturateOnIntegerOverflow=off  RndMeth=Floor
  Delay{59..63,65..71} (12 alike) : Delay  DelayLength=1  InitialCondition=0
  Product3 : Product  OutDataTypeStr=int64
  Shift Arithmetic2 : ArithShift  BitShiftNumberSource=Input port  BitShiftNumber=8  BitShiftDirection=Left
      settings: InputPortMap=u0,p1
  Shift Arithmetic3 : ArithShift  BitShiftNumberSource=Input port  BitShiftNumber=8  BitShiftDirection=Left
      settings: InputPortMap=u0,p1
  Sum1 : Sum  Inputs=|++  OutDataTypeStr=int64
  Sum3 : Sum  Inputs=|+-  OutDataTypeStr=int64
  Sum4 : Sum  Inputs=|+-  OutDataTypeStr=int64
  Sum5 : Sum  Inputs=|++  OutDataTypeStr=int64
  const1 : Constant  OutDataTypeStr=int64  SampleTime=t_clock
  const3 : Constant  OutDataTypeStr=int64  SampleTime=t_clock
  const5 : Constant  OutDataTypeStr=int64  SampleTime=t_clock
  floor_div_pow2 : Subsystem
  st_raw_with_offset_and_wrapped : Outport  SampleTime=1e-08
  mt_raw_with_offset_and_wrapped : Outport  Port=2  SampleTime=1e-08
  wires:
  Delay69/1 -> Sum1/2
  Delay60/1 -> Delay67/1, Product3/2
  Delay61/1 -> Delay68/1
  mt_raw/1 -> Data Type Conversion3/1
  Shift Arithmetic3/1 -> Delay60/1
  const5/1 -> Shift Arithmetic3/1
  Data Type Conversion6/1 -> mt_raw_with_offset_and_wrapped/1
  n/1 -> Delay61/1, Shift Arithmetic3/2
  Data Type Conversion4/1 -> Delay62/1
  Data Type Conversion3/1 -> Delay59/1
  st_raw/1 -> Data Type Conversion4/1
  Sum4/1 -> Bitwise AND2/2
  Delay59/1 -> Product3/1
  In4/1 -> Data Type Conversion2/1
  Product3/1 -> Delay66/1
  Sum1/1 -> Sum5/1
  Delay62/1 -> Delay69/1
  const3/1 -> Shift Arithmetic2/1
  Data Type Conversion2/1 -> Delay63/1
  n1/1 -> Shift Arithmetic2/2
  Delay67/1 -> Sum3/1
  Delay66/1 -> Sum1/1
  Sum3/1 -> Bitwise AND3/2
  Delay63/1 -> Delay70/1
  Shift Arithmetic2/1 -> Delay65/1
  Delay70/1 -> Sum5/2
  const1/1 -> Sum3/2, Sum4/2
  Delay65/1 -> Delay71/1
  Sum5/1 -> Bitwise AND3/1, floor_div_pow2/1(dividend)
  Delay68/1 -> floor_div_pow2/2(divisor_power_of_two_bits)
  Delay71/1 -> Sum4/1
  Bitwise AND3/1 -> Data Type Conversion5/1
  floor_div_pow2/1(quotient) -> Bitwise AND2/1
  Data Type Conversion5/1 -> st_raw_with_offset_and_wrapped/1
  Bitwise AND2/1 -> Data Type Conversion6/1

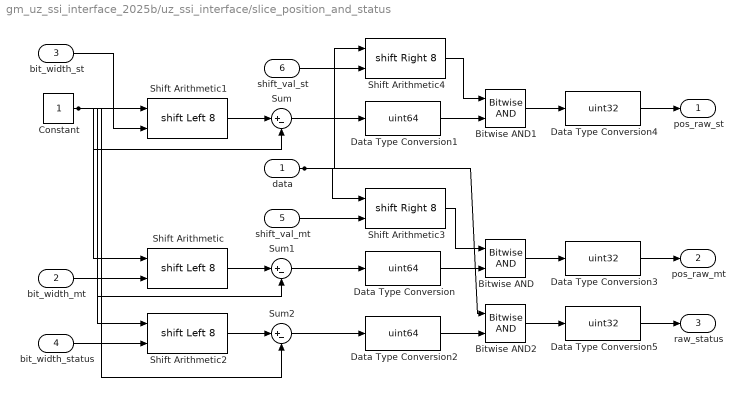
== system gm_uz_ssi_interface_2025b/uz_ssi_interface/slice_position_and_status ==
  data : Inport  OutDataTypeStr=fixdt(0, 64, 0)  PortDimensions=1  SampleTime=1e-08
  bit_width_mt : Inport  Port=2  OutDataTypeStr=uint32  PortDimensions=1  SampleTime=1e-08
  bit_width_st : Inport  Port=3  OutDataTypeStr=uint32  PortDimensions=1  SampleTime=1e-08
  bit_width_status : Inport  Port=4  OutDataTypeStr=uint32  PortDimensions=1  SampleTime=1e-08
  shift_val_mt : Inport  Port=5  OutDataTypeStr=int32  PortDimensions=1  SampleTime=1e-08
  shift_val_st : Inport  Port=6  OutDataTypeStr=int32  PortDimensions=1  SampleTime=1e-08
  Bitwise AND : simulink/Logic and Bit Operations/Bitwise Operator  logicop=AND  UseBitMask=off  NumInputPorts=2  BitMask=bin2dec('11011001')  BitMaskRealWorld=Stored Integer
      settings: LibrarySourceBlock=|
      | simulink/Quick Insert/Logic and Bit
      | Operations/Bitwise AND
  Bitwise AND1 : simulink/Logic and Bit Operations/Bitwise Operator  logicop=AND  UseBitMask=off  NumInputPorts=2  BitMask=bin2dec('11011001')  BitMaskRealWorld=Stored Integer
      settings: LibrarySourceBlock=|
      | simulink/Quick Insert/Logic and Bit
      | Operations/Bitwise AND
  Bitwise AND2 : simulink/Logic and Bit Operations/Bitwise Operator  logicop=AND  UseBitMask=off  NumInputPorts=2  BitMask=bin2dec('11011001')  BitMaskRealWorld=Stored Integer
      settings: LibrarySourceBlock=|
      | simulink/Quick Insert/Logic and Bit
      | Operations/Bitwise AND
  Constant : Constant  OutDataTypeStr=uint32  SampleTime=t_clock
  Data Type Conversion : DataTypeConversion  OutDataTypeStr=uint64  SaturateOnIntegerOverflow=off  RndMeth=Floor
  Data Type Conversion1 : DataTypeConversion  OutDataTypeStr=uint64  SaturateOnIntegerOverflow=off  RndMeth=Floor
  Data Type Conversion2 : DataTypeConversion  OutDataTypeStr=uint64  SaturateOnIntegerOverflow=off  RndMeth=Floor
  Data Type Conversion3 : DataTypeConversion  OutDataTypeStr=uint32  SaturateOnIntegerOverflow=off  RndMeth=Floor
  Data Type Conversion4 : DataTypeConversion  OutDataTypeStr=uint32  SaturateOnIntegerOverflow=off  RndMeth=Floor
  Data Type Conversion5 : DataTypeConversion  OutDataTypeStr=uint32  SaturateOnIntegerOverflow=off  RndMeth=Floor
  Shift Arithmetic : ArithShift  BitShiftNumberSource=Input port  BitShiftNumber=8  BitShiftDirection=Left
      settings: InputPortMap=u0,p1
  Shift Arithmetic1 : ArithShift  BitShiftNumberSource=Input port  BitShiftNumber=8  BitShiftDirection=Left
      settings: InputPortMap=u0,p1
  Shift Arithmetic2 : ArithShift  BitShiftNumberSource=Input port  BitShiftNumber=8  BitShiftDirection=Left
      settings: InputPortMap=u0,p1
  Shift Arithmetic3 : ArithShift  BitShiftNumberSource=Input port  BitShiftNumber=8  BitShiftDirection=Right
      settings: InputPortMap=u0,p1
  Shift Arithmetic4 : ArithShift  BitShiftNumberSource=Input port  BitShiftNumber=8  BitShiftDirection=Right
      settings: InputPortMap=u0,p1
  Sum : Sum  Inputs=|+-  OutDataTypeStr=uint32
  Sum1 : Sum  Inputs=|+-  OutDataTypeStr=uint32
  Sum2 : Sum  Inputs=|+-  OutDataTypeStr=uint32
  pos_raw_st : Outport  SampleTime=1e-08
  pos_raw_mt : Outport  Port=2  SampleTime=1e-08
  raw_status : Outport  Port=3  SampleTime=1e-08
  wires:
  shift_val_mt/1 -> Shift Arithmetic3/2
  shift_val_st/1 -> Shift Arithmetic4/2
  Data Type Conversion5/1 -> raw_status/1
  bit_width_st/1 -> Shift Arithmetic1/2
  Constant/1 -> Sum2/2, Sum1/2, Sum/2, Shift Arithmetic1/1, Shift Arithmetic2/1, Shift Arithmetic/1
  Shift Arithmetic2/1 -> Sum2/1
  bit_width_mt/1 -> Shift Arithmetic/2
  bit_width_status/1 -> Shift Arithmetic2/2
  Shift Arithmetic1/1 -> Sum/1
  Shift Arithmetic/1 -> Sum1/1
  Sum/1 -> Data Type Conversion1/1
  data/1 -> Bitwise AND2/1, Shift Arithmetic4/1, Shift Arithmetic3/1
  Sum1/1 -> Data Type Conversion/1
  Sum2/1 -> Data Type Conversion2/1
  Shift Arithmetic4/1 -> Bitwise AND1/1
  Data Type Conversion2/1 -> Bitwise AND2/2
  Data Type Conversion1/1 -> Bitwise AND1/2
  Bitwise AND/1 -> Data Type Conversion3/1
  Shift Arithmetic3/1 -> Bitwise AND/1
  Data Type Conversion/1 -> Bitwise AND/2
  Bitwise AND1/1 -> Data Type Conversion4/1
  Bitwise AND2/1 -> Data Type Conversion5/1
  Data Type Conversion4/1 -> pos_raw_st/1
  Data Type Conversion3/1 -> pos_raw_mt/1

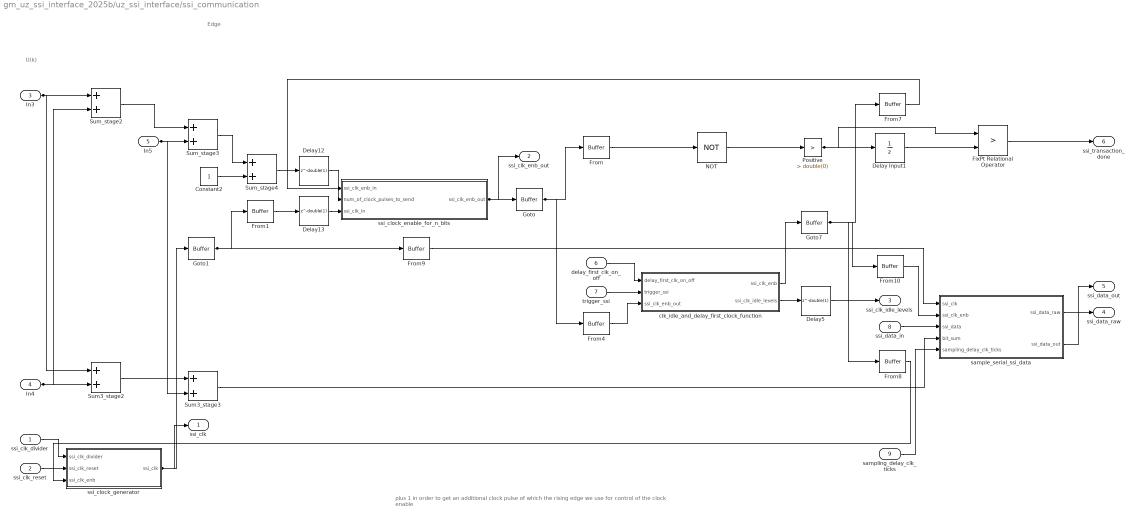
== system gm_uz_ssi_interface_2025b/uz_ssi_interface/ssi_communication ==
  note: U(k)
  note: Edge
  note: plus 1 in order to get an additional clock pulse of which the rising edge we use for control of the clock enable
  ssi_clk_divider : Inport  OutDataTypeStr=uint32  PortDimensions=1  SampleTime=1e-08
  ssi_clk_reset : Inport  Port=2  OutDataTypeStr=boolean  PortDimensions=1  SampleTime=1e-08
  In3 : Inport  Port=3  OutDataTypeStr=uint32  PortDimensions=1  SampleTime=1e-08
  In4 : Inport  Port=4  OutDataTypeStr=uint32  PortDimensions=1  SampleTime=1e-08
  In5 : Inport  Port=5  OutDataTypeStr=uint32  PortDimensions=1  SampleTime=1e-08
  delay_first_clk_on_off : Inport  Port=6  OutDataTypeStr=boolean  PortDimensions=1  SampleTime=1e-08
  trigger_ssi : Inport  Port=7  OutDataTypeStr=boolean  PortDimensions=1  SampleTime=1e-08
  ssi_data_in : Inport  Port=8  OutDataTypeStr=boolean  PortDimensions=1  SampleTime=1e-08
  sampling_delay_clk_ticks : Inport  Port=9  OutDataTypeStr=uint32  PortDimensions=1  SampleTime=1e-08
  Constant2 : Constant  OutDataTypeStr=uint32  SampleTime=1e-08
  Delay Input1 : UnitDelay  SampleTime=1e-08
  Delay12 : Delay  DelayLength=double(1)  InitialCondition=0  SampleTime=1e-08
  Delay13 : Delay  DelayLength=double(1)  InitialCondition=0  SampleTime=1e-08
  Delay5 : Delay  DelayLength=double(1)  InitialCondition=0  SampleTime=1e-08
  FixPt Relational Operator : RelationalOperator  Operator=>  OutDataTypeStr=boolean  SampleTime=1e-08  InputSameDT=off
  From{,1,4,7..10} (7 alike) : hdlmdlgenlib/Buffer
  Goto : hdlmdlgenlib/Buffer
  Goto1 : hdlmdlgenlib/Buffer
  Goto7 : hdlmdlgenlib/Buffer
  NOT : Logic  Operator=NOT  Inputs=1  AllPortsSameDT=off  OutDataTypeStr=boolean  SampleTime=1e-08
  Positive : simulink/Logic and Bit Operations/Compare To Constant  relop=>  const=double(0)  OutDataTypeStr=boolean
  Sum3_stage2 : Sum  OutDataTypeStr=fixdt(0, 33, 0)  AccumDataTypeStr=uint32  SampleTime=1e-08
  Sum3_stage3 : Sum  OutDataTypeStr=uint32  AccumDataTypeStr=uint32  SampleTime=1e-08
  Sum_stage2 : Sum  OutDataTypeStr=fixdt(0, 33, 0)  AccumDataTypeStr=uint32  SampleTime=1e-08
  Sum_stage3 : Sum  OutDataTypeStr=fixdt(0, 34, 0)  AccumDataTypeStr=uint32  SampleTime=1e-08
  Sum_stage4 : Sum  OutDataTypeStr=uint32  AccumDataTypeStr=uint32  SampleTime=1e-08
  clk_idle_and_delay_first_clock_function : Subsystem
  sample_serial_ssi_data : Subsystem
  ssi_clock_enable_for_n_bits : Subsystem
  ssi_clock_generator : Subsystem
  ssi_clk : Outport  SampleTime=1e-08
  ssi_clk_enb_out : Outport  Port=2  SampleTime=1e-08
  ssi_clk_idle_levels : Outport  Port=3  SampleTime=1e-08
  ssi_data_raw : Outport  Port=4  SampleTime=1e-08
  ssi_data_out : Outport  Port=5  SampleTime=1e-08
  ssi_transaction_done : Outport  Port=6  SampleTime=1e-08
  wires:
  clk_idle_and_delay_first_clock_function/2(ssi_clk_idle_levels) -> Delay5/1
  In3/1 -> Sum3_stage2/1, Sum_stage2/1
  From9/1 -> sample_serial_ssi_data/1(ssi_clk)
  Sum_stage4/1 -> Delay12/1
  In4/1 -> Sum3_stage2/2, Sum_stage2/2
  In5/1 -> Sum3_stage3/2, Sum_stage3/2
  ssi_clk_divider/1 -> ssi_clock_generator/1(ssi_clk_divider)
  sample_serial_ssi_data/1(ssi_data_raw) -> ssi_data_raw/1
  ssi_clk_reset/1 -> ssi_clock_generator/2(ssi_clk_reset)
  Sum_stage2/1 -> Sum_stage3/1
  delay_first_clk_on_off/1 -> clk_idle_and_delay_first_clock_function/1(delay_first_clk_on_off)
  Sum3_stage2/1 -> Sum3_stage3/1
  ssi_clock_generator/1(ssi_clk) -> ssi_clk/1, Goto1/1
  sample_serial_ssi_data/2(ssi_data_out) -> ssi_data_out/1
  Sum_stage3/1 -> Sum_stage4/1
  Constant2/1 -> Sum_stage4/2
  FixPt Relational Operator/1 -> ssi_transaction_done/1
  trigger_ssi/1 -> clk_idle_and_delay_first_clock_function/2(trigger_ssi)
  Goto1/1 -> From9/1, From1/1
  Sum3_stage3/1 -> sample_serial_ssi_data/4(bit_sum)
  From1/1 -> Delay13/1
  Delay12/1 -> ssi_clock_enable_for_n_bits/2(num_of_clock_pulses_to_send)
  Delay13/1 -> ssi_clock_enable_for_n_bits/3(ssi_clk_in)
  ssi_clock_enable_for_n_bits/1(ssi_clk_enb_out) -> ssi_clk_enb_out/1, Goto/1
  Goto/1 -> From/1, From4/1
  From/1 -> NOT/1
  From4/1 -> clk_idle_and_delay_first_clock_function/3(ssi_clk_enb_out)
  Delay Input1/1 -> FixPt Relational Operator/2
  From7/1 -> ssi_clock_enable_for_n_bits/1(ssi_clk_enb_in)
  NOT/1 -> Positive/1
  clk_idle_and_delay_first_clock_function/1(ssi_clk_enb) -> Goto7/1
  Positive/1 -> FixPt Relational Operator/1, Delay Input1/1
  Goto7/1 -> From7/1, From8/1, From10/1
  Delay5/1 -> ssi_clk_idle_levels/1
  From10/1 -> sample_serial_ssi_data/2(ssi_clk_enb)
  sampling_delay_clk_ticks/1 -> sample_serial_ssi_data/5(sampling_delay_clk_ticks)
  ssi_data_in/1 -> sample_serial_ssi_data/3(ssi_data)
  From8/1 -> ssi_clock_generator/3(ssi_clk_enb)

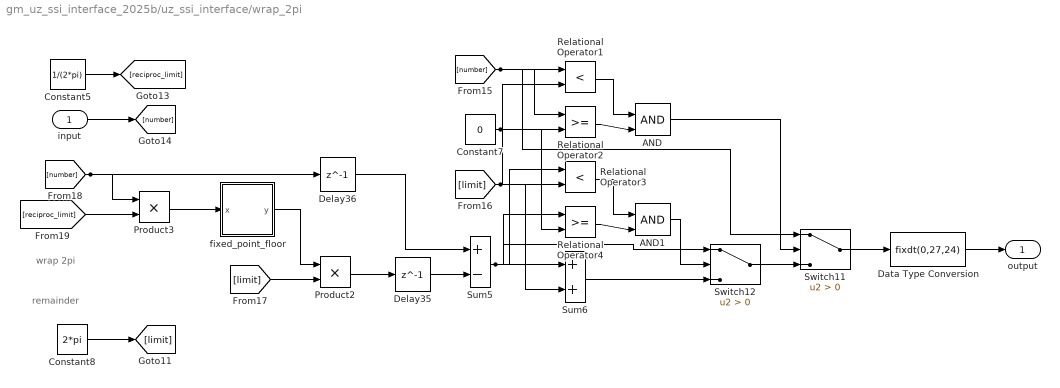
== system gm_uz_ssi_interface_2025b/uz_ssi_interface/wrap_2pi ==
  note: remainder
  note: wrap 2pi
  input : Inport  OutDataTypeStr=fixdt(0, 27, 20)  PortDimensions=1  SampleTime=1e-08
  AND : Logic  IconShape=distinctive  AllPortsSameDT=off  OutDataTypeStr=boolean
  AND1 : Logic  IconShape=distinctive  AllPortsSameDT=off  OutDataTypeStr=boolean
  Constant5 : Constant  Value=1/(2*pi)  OutDataTypeStr=fixdt(0,18,20)  SampleTime=-1
  Constant7 : Constant  Value=0  OutDataTypeStr=fixdt(0,27,24)  SampleTime=-1
  Constant8 : Constant  Value=2*pi  OutDataTypeStr=fixdt(0,18,15)  SampleTime=-1
  Data Type Conversion : DataTypeConversion  OutDataTypeStr=fixdt(0,27,24)  SaturateOnIntegerOverflow=off  RndMeth=Floor
  Delay35 : Delay  DelayLength=1  InitialCondition=0
  Delay36 : Delay  DelayLength=1  InitialCondition=0
  Product2 : Product  OutDataTypeStr=fixdt(0,27,24)
  Product3 : Product  OutDataTypeStr=fixdt(0,27,24)
  Relational Operator1 : RelationalOperator  Operator=<  OutDataTypeStr=boolean  RndMeth=Simplest  InputSameDT=off
  Relational Operator2 : RelationalOperator  OutDataTypeStr=boolean  RndMeth=Simplest  InputSameDT=off
  Relational Operator3 : RelationalOperator  Operator=<  OutDataTypeStr=boolean  RndMeth=Simplest  InputSameDT=off
  Relational Operator4 : RelationalOperator  OutDataTypeStr=boolean  RndMeth=Simplest  InputSameDT=off
  Sum5 : Sum  Inputs=+-  OutDataTypeStr=fixdt(0,27,24)
  Sum6 : Sum  OutDataTypeStr=fixdt(0,27,24)
  Switch11 : Switch  Criteria=u2 > Threshold  OutDataTypeStr=fixdt(0, 27, 20)  SaturateOnIntegerOverflow=off  InputSameDT=off
  Switch12 : Switch  Criteria=u2 > Threshold  OutDataTypeStr=fixdt(0, 27, 24)  SaturateOnIntegerOverflow=off  InputSameDT=off
  fixed_point_floor : Subsystem
  output : Outport  SampleTime=1e-08
  wires:
  input/1 -> [number]
  Constant5/1 -> [reciproc_limit]
  Data Type Conversion/1 -> output/1
  [number] -> Product3/1, Delay36/1
  [limit] -> Product2/2
  [reciproc_limit] -> Product3/2
  Constant8/1 -> [limit]
  Product3/1 -> fixed_point_floor/1(x)
  fixed_point_floor/1(y) -> Product2/1
  Relational Operator2/1 -> AND/2
  Delay36/1 -> Sum5/1
  Product2/1 -> Delay35/1
  Delay35/1 -> Sum5/2
  Relational Operator3/1 -> AND1/1
  [limit] -> Sum6/2, Relational Operator3/2, Relational Operator1/2
  [number] -> Switch11/1, Relational Operator2/1, Relational Operator1/1
  Constant7/1 -> Relational Operator4/2, Relational Operator2/2
  Sum5/1 -> Sum6/1, Relational Operator4/1, Relational Operator3/1, Switch12/1
  Relational Operator1/1 -> AND/1
  Relational Operator4/1 -> AND1/2
  Sum6/1 -> Switch12/3
  AND/1 -> Switch11/2
  AND1/1 -> Switch12/2
  Switch12/1 -> Switch11/3
  Switch11/1 -> Data Type Conversion/1
